simulink model "Full_Wave_Controlled_Rectifier"  (R2023b)
settings: Solver=VariableStepAuto  StartTime=0.0  StopTime=1  RelTol=1e-3
undefined symbols (not defined in the file): a
libraries: spsThyristorLib x4, spsACVoltageSourceLib x1, spsMultimeterLib x1, spsSeriesRLCBranchLib x1, sps_lib x1
settings Model: Creator=HP  LastModifiedBy=HP

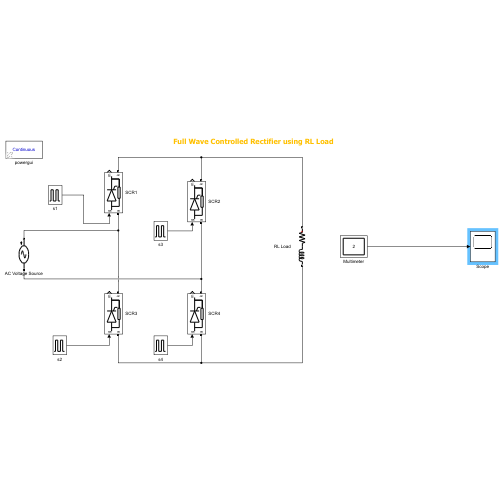
[thumbnail: Simulink's stored preview of the top-level diagram]
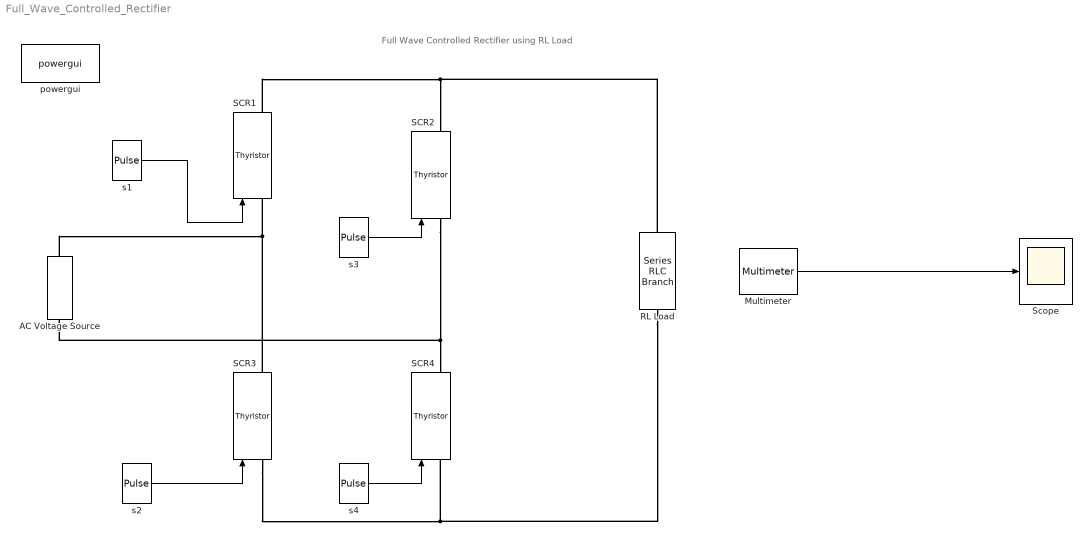
== system Full_Wave_Controlled_Rectifier ==
  note: Full Wave Controlled Rectifier using RL Load
  AC Voltage Source : spsACVoltageSourceLib/AC Voltage Source  Amplitude=320  Phase=0  Frequency=50  SampleTime=0  Measurements=Voltage  BusType=swing  Pref=10e3  Qref=0  Qmin=-inf  Qmax=+inf
  Multimeter : spsMultimeterLib/Multimeter  L=2  sel=[2 1]  yselected={}  Gain=[1 1]  OutputType=Complex  PlotAtSimulationStop=off  PhasorSimulation=off
  RL Load : spsSeriesRLCBranchLib/Series RLC Branch  LConnTagsString=__new0  RConnTagsString=__new0  BranchType=RL  Resistance=10  Inductance=5e-3  SetiL0=off  InitialCurrent=0  Capacitance=1e-6  Setx0=off  InitialVoltage=0  Measurements=Branch voltage
  SCR{1..4} (4 alike) : spsThyristorLib/Thyristor  Ron=0.001  Lon=0  Vf=0.8  IC=0  Rs=500  Cs=250e-9  Measurements=on
  Scope : Scope
  powergui : sps_lib/powergui  Priority=1  SimulationMode=Continuous  SampleTime=50e-6  frequency=60  Iterations=50  frequencyindice=50  Pbase=100e6  ErrMax=1e-4  UnitsV=kV  UnitsW=MW  buscounter=0  FunctionMessages=off  echomessages=off  EnableUseOfTLC=off  CurrentSourceSwitches=off  DisableSnubberDevices=off  DisableRonSwitches=off  DisableVfSwitches=off  DisplayEquations=off  AutomaticDiscreteSolvers=off  SolverType=Tustin/Backward Euler (TBE)  Interpol=off  ExternalGateDelay=off  methode=off  Ts=100  x0status=blocks  SPID=on  SwTol=0  HookPort=off  NonlinearTolerance=1e-4  nMaxIteration=100  ContinueOnMaxIteration=off  RestoreLinks=warning  ResistiveCurrentMeasurement=off  Frange=[0:2:500]  Ylog=off  Xlog=on  ShowGrid=off  save=off  variable=ZData  structure=0  ZoomFFT=off  StartTime=0.0  cycles=1  DisplayStyle=1  fundamental=60  FreqAxis=off  MaxFrequency=1000  frequencyindicesteady=1  RmsSteady=1  display=off
  s1 : DiscretePulseGenerator  PulseType=Time based  Period=1/50  PulseWidth=5  PhaseDelay=a*0.02/360
  s2 : DiscretePulseGenerator  PulseType=Time based  Period=1/50  PulseWidth=5  PhaseDelay=(a+180)*0.02/360
  s3 : DiscretePulseGenerator  PulseType=Time based  Period=1/50  PulseWidth=5  PhaseDelay=(a+180)*0.02/360
  s4 : DiscretePulseGenerator  PulseType=Time based  Period=1/50  PulseWidth=5  PhaseDelay=a*0.02/360
  wires:
  s1/1 -> SCR1/1
  s2/1 -> SCR3/1
  s3/1 -> SCR2/1
  s4/1 -> SCR4/1
  Multimeter/1 -> Scope/1
  connections:
  SCR3/RConn1 -- AC Voltage Source/RConn1 -- SCR1/LConn1
  SCR1/RConn1 -- RL Load/LConn1 -- SCR2/RConn1
  SCR3/LConn1 -- SCR4/LConn1 -- RL Load/RConn1
  SCR2/LConn1 -- SCR4/RConn1 -- AC Voltage Source/LConn1
